simulink model "ejemplo_3_lazo_cerrado_router"  (R2026a)
settings: Solver=FixedStepAuto  StopTime=inf
libraries: ros2lib x4
settings Model: Creator=samuel  LastModifiedBy=samuelpz
settings HardwareCC: ProdBitPerLong=64.0  ProdHWDeviceType=Intel->x86-64 (Linux 64)  UseEmbeddedCoderFeatures=off
settings RTWCC: SystemTargetFile=ert.tlc  HardwareBoard=Robot Operating System 2 (ROS 2)  TLCOptions="-aInlineSetEventsForThisBaseRateFcn=TLC_FALSE -aSuppressMultiTaskScheduler=TLC_FALSE  -aRateBasedStepFcn=0"  Toolchain=Colcon Tools  TargetLang=C++  Description=Embedded Coder
settings ERTTargetCC: ExtModeTransport=2.0  ExtModeAutomaticAllocSize=off  RootIOFormat=Structure reference  CodeInterfacePackaging=C++ class  SupportNonInlinedSFcns=on

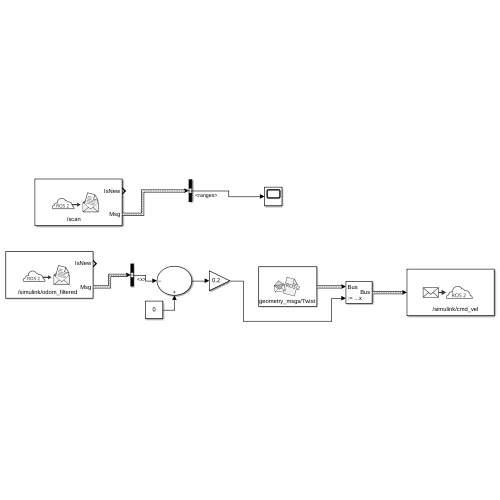
[thumbnail: Simulink's stored preview of the top-level diagram]
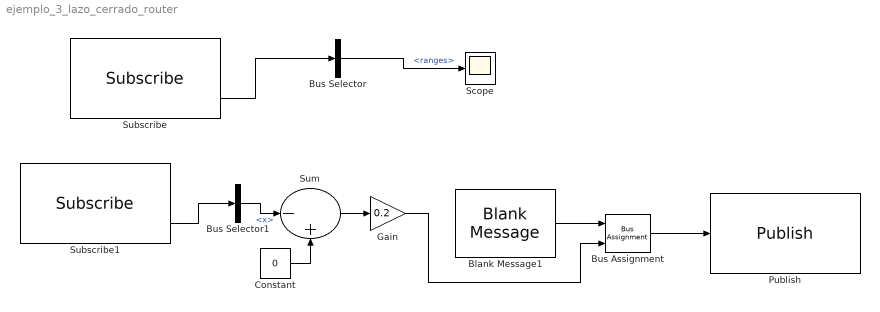
== system ejemplo_3_lazo_cerrado_router ==
  Blank Message1 : ros2lib/Blank Message  messageClass=Message  entityType=geometry_msgs/Twist  messageType=geometry_msgs/Twist  SampleTime=inf
  Bus Assignment : BusAssignment  AssignedSignals=linear.x
  Bus Selector : BusSelector  OutputSignals=ranges
  Bus Selector1 : BusSelector  OutputSignals=pose.pose.position.x
  Constant : Constant  Value=0
  Gain : Gain  Gain=0.2
  Publish : ros2lib/Publish  topicSource=Specify your own  topic=/simulink/cmd_vel  messageType=geometry_msgs/Twist  QOSHistory=Keep last  QOSDepth=10  QOSReliability=Reliable  QOSDurability=Volatile  QOSDeadline=Inf  QOSLifespan=Inf  QOSLiveliness=Automatic  QOSLeaseDuration=Inf  QOSAvoidROSNamespaceConventions=off
  Scope : Scope
      settings: ActiveDisplayYMinimum=-3.4084929327100788  ActiveDisplayYMaximum=11.193974313618298
  Subscribe : ros2lib/Subscribe  topicSource=Specify your own  topic=/scan  messageType=sensor_msgs/LaserScan  sampleTime=-1  QOSHistory=Keep last  QOSDepth=10  QOSReliability=Reliable  QOSDurability=Volatile  QOSDeadline=Inf  QOSLifespan=Inf  QOSLiveliness=Automatic  QOSLeaseDuration=Inf  QOSAvoidROSNamespaceConventions=off
  Subscribe1 : ros2lib/Subscribe  topicSource=Specify your own  topic=/simulink/odom_filtered  messageType=nav_msgs/Odometry  sampleTime=-1  QOSHistory=Keep last  QOSDepth=10  QOSReliability=Reliable  QOSDurability=Volatile  QOSDeadline=Inf  QOSLifespan=Inf  QOSLiveliness=Automatic  QOSLeaseDuration=Inf  QOSAvoidROSNamespaceConventions=off
  Sum : Sum  Inputs=|-+
  wires:
  Bus Selector/1 -> Scope/1  "<ranges>"
  Constant/1 -> Sum/2
  Sum/1 -> Gain/1
  Blank Message1/1 -> Bus Assignment/1
  Gain/1 -> Bus Assignment/2
  Bus Assignment/1 -> Publish/1
  Subscribe/2 -> Bus Selector/1
  Subscribe1/2 -> Bus Selector1/1
  Bus Selector1/1 -> Sum/1  "<x>"
